simulink model "chirp2"  (R2024a)
settings: Solver=FixedStepDiscrete  StartTime=0.0  StopTime=0.001024  FixedStep=0.00000005  RelTol=1e-3
libraries: simulink x2, dspstat3 x2, dspswit3 x1, dspxfrm3 x1, commrandsrc3 x1
settings Model: Creator=Varun Prasath R
settings ConfigComp: CovBoundaryAbsTol=1.0e-5

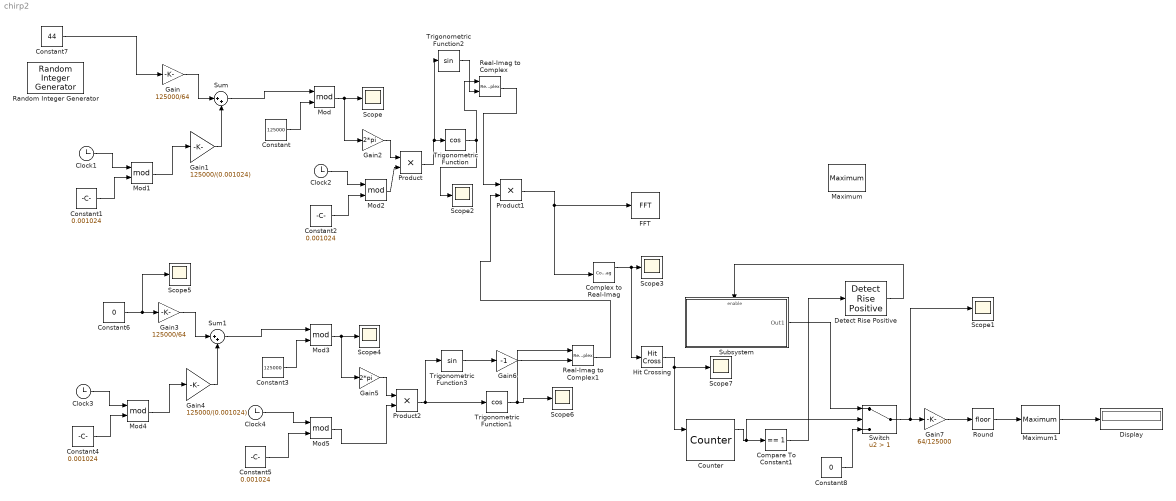
== system chirp2 ==
  Clock{1..4} (4 alike) : Clock
  Compare To Constant1 : simulink/Logic and Bit Operations/Compare To Constant  relop===  const=1  OutDataTypeStr=boolean
  Complex to Real-Imag : ComplexToRealImag
  Constant : Constant  Value=125000
  Constant{1..2,4..5} (4 alike) : Constant  Value=0.001024
  Constant3 : Constant  Value=125000
  Constant6 : Constant  Value=0
  Constant7 : Constant  Value=44
  Constant8 : Constant  Value=0
  Counter : dspswit3/Counter  Direction=Up  CountEvent=Rising edge  CounterSize=User defined  MaxCount=255  InitialCount=0  Output=Count and Hit  HitValue=32  ResetInput=on  SamplesPerFrame=1  Ts=1  CntDtype=double  HitDtype=Logical
  Detect Rise Positive : simulink/Logic and Bit Operations/Detect Rise Positive  vinit=0  OutDataTypeStr=boolean
  Display : Display
  FFT : dspxfrm3/FFT  FFTImplementation=Auto  CompMethod=Table lookup  TableOpt=NEW  TableOptActive=Speed  BitRevOrder=off  Normalize=off  InheritFFTLength=on  FFTLength=1000  WrapInput=off  roundingMode=Ceiling  overflowMode=off  firstCoeffDataTypeStr=Inherit: Same word length as input  firstCoeffLastDataTypeStr=Inherit: Same word length as input  outputMin=[]  outputMax=[]
  Gain : Gain  Gain=125000/64
  Gain1 : Gain  Gain=125000/(0.001024)
  Gain2 : Gain  Gain=2*pi
  Gain3 : Gain  Gain=125000/64
  Gain4 : Gain  Gain=125000/(0.001024)
  Gain5 : Gain  Gain=2*pi
  Gain6 : Gain  Gain=-1
  Gain7 : Gain  Gain=64/125000
  Hit Crossing : HitCross  HitCrossingOffset=0.999  HitCrossingDirection=rising
  Maximum : dspstat3/Maximum  operation=maximum  fcn=Value and Index  indexBase=One  operateOver=Each column  Dimension=1  InputProcessing=Columns as channels (frame based)  reset=None  roiEnable=off  roiType=Rectangles  roiPortion=Entire ROI  roiOutput=Individual statistics for each ROI  roiFlag=off  roundingMode=Floor  overflowMode=off  accumDataTypeStr=Inherit: Same as product output  accumLastDataTypeStr=Inherit: Same as product output
  Maximum1 : dspstat3/Maximum  operation=maximum  fcn=Running  indexBase=One  operateOver=Each column  Dimension=1  InputProcessing=Columns as channels (frame based)  reset=None  roiEnable=off  roiType=Rectangles  roiPortion=Entire ROI  roiOutput=Individual statistics for each ROI  roiFlag=off  roundingMode=Floor  overflowMode=off  accumDataTypeStr=Inherit: Same as product output  accumLastDataTypeStr=Inherit: Same as product output
  Mod{,1..5} (6 alike) : Math  Operator=mod
  Product : Product
  Product1 : Product
  Product2 : Product
  Random Integer Generator : commrandsrc3/Random Integer Generator  SetSize=128  SeedSource=Auto  Seed=0  SampleTime=0.001024  SamplesPerFrame=1  OutputDataType=double  SimulateUsing=Interpreted execution
  Real-Imag to Complex : RealImagToComplex
  Real-Imag to Complex1 : RealImagToComplex
  Round : Rounding
  Scope{,1..7} (8 alike) : Scope
  Subsystem : Subsystem
  Sum : Sum  Inputs=|++
  Sum1 : Sum  Inputs=|++
  Switch : Switch  Criteria=u2 > Threshold  Threshold=1  SaturateOnIntegerOverflow=off  InputSameDT=off
  Trigonometric Function : Trigonometry  Operator=cos
  Trigonometric Function1 : Trigonometry  Operator=cos
  Trigonometric Function2 : Trigonometry
  Trigonometric Function3 : Trigonometry
  wires:
  Constant/1 -> Mod/2
  Mod/1 -> Gain2/1, Scope/1
  Mod1/1 -> Gain1/1
  Constant1/1 -> Mod1/2
  Clock1/1 -> Mod1/1
  Gain/1 -> Sum/1
  Gain1/1 -> Sum/2
  Sum/1 -> Mod/1
  Trigonometric Function/1 -> Real-Imag to Complex/1, Scope2/1
  Clock2/1 -> Mod2/1
  Constant2/1 -> Mod2/2
  Gain2/1 -> Product/1
  Mod2/1 -> Product/2
  Product/1 -> Trigonometric Function2/1, Trigonometric Function/1
  Trigonometric Function1/1 -> Real-Imag to Complex1/1, Scope6/1
  Mod4/1 -> Gain4/1
  Mod3/1 -> Gain5/1, Scope4/1
  Constant6/1 -> Scope5/1, Gain3/1
  Constant3/1 -> Mod3/2
  Sum1/1 -> Mod3/1
  Gain4/1 -> Sum1/2
  Clock3/1 -> Mod4/1
  Gain3/1 -> Sum1/1
  Gain5/1 -> Product2/1
  Constant5/1 -> Mod5/2
  Constant4/1 -> Mod4/2
  Clock4/1 -> Mod5/1
  Mod5/1 -> Product2/2
  Trigonometric Function2/1 -> Real-Imag to Complex/2
  Real-Imag to Complex1/1 -> Product1/2
  Product2/1 -> Trigonometric Function1/1, Trigonometric Function3/1
  Trigonometric Function3/1 -> Gain6/1
  Gain6/1 -> Real-Imag to Complex1/2
  Real-Imag to Complex/1 -> Product1/1
  Constant7/1 -> Gain/1
  Product1/1 -> Complex to Real-Imag/1, FFT/1
  Complex to Real-Imag/1 -> Scope3/1, Hit Crossing/1
  Hit Crossing/1 -> Counter/1, Scope7/1
  Subsystem/1(Out1) -> Switch/1
  Constant8/1 -> Switch/3
  Switch/1 -> Scope1/1, Gain7/1
  Gain7/1 -> Round/1
  Round/1 -> Maximum1/1
  Maximum1/1 -> Display/1
  Counter/1 -> Compare To Constant1/1, Switch/2
  Compare To Constant1/1 -> Detect Rise Positive/1
  Detect Rise Positive/1 -> Subsystem/Enable

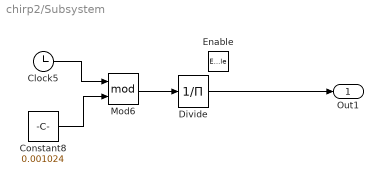
== system chirp2/Subsystem ==
  Enable : EnablePort
  Clock5 : Clock
  Constant8 : Constant  Value=0.001024
  Divide : Product  Inputs=/
  Mod6 : Math  Operator=mod
  Out1 : Outport
  wires:
  Clock5/1 -> Mod6/1
  Constant8/1 -> Mod6/2
  Mod6/1 -> Divide/1
  Divide/1 -> Out1/1
